simulink model "aaaqi"  (R2016b)
settings: Solver=ode4  StartTime=0.0  StopTime=inf  FixedStep=0.002  RelTol=1e-3  EnableMultiTasking=on
undefined symbols (not defined in the file or in its folder): bit, mdaadlink6208, sigbuilder_block, Standard
libraries: slrtlib x20, slrtsoftinglib x11, simulink x10
(part 1 of 4)
settings Model: xpc_rtwmakecfg_data=_xpccanac2pci_  SimulationMode=external  Creator=Administrator  LastModifiedBy=Administrator
settings SolverCC: EnableConcurrentExecution=on
settings DataIOCC: SaveFormat=StructureWithTime
settings OptimizationCC: BlockReduction=off  OptimizeBlockIOStorage=off  BufferReuse=off  GlobalBufferReuse=off  ExpressionFolding=off  LocalBlockOutputs=off
settings HardwareCC: ProdBitPerPointer=32  ProdBitPerSizeT=32  ProdBitPerPtrDiffT=32  ProdLargestAtomicFloat=None  ProdWordSize=32  ProdLongLongMode=on  ProdHWDeviceType=Generic->32-bit x86 compatible
settings RTWCC: SystemTargetFile=slrt.tlc  TemplateMakefile=slrt_default_tmf  Description=Simulink Real-Time  RTWCompilerOptimization=on

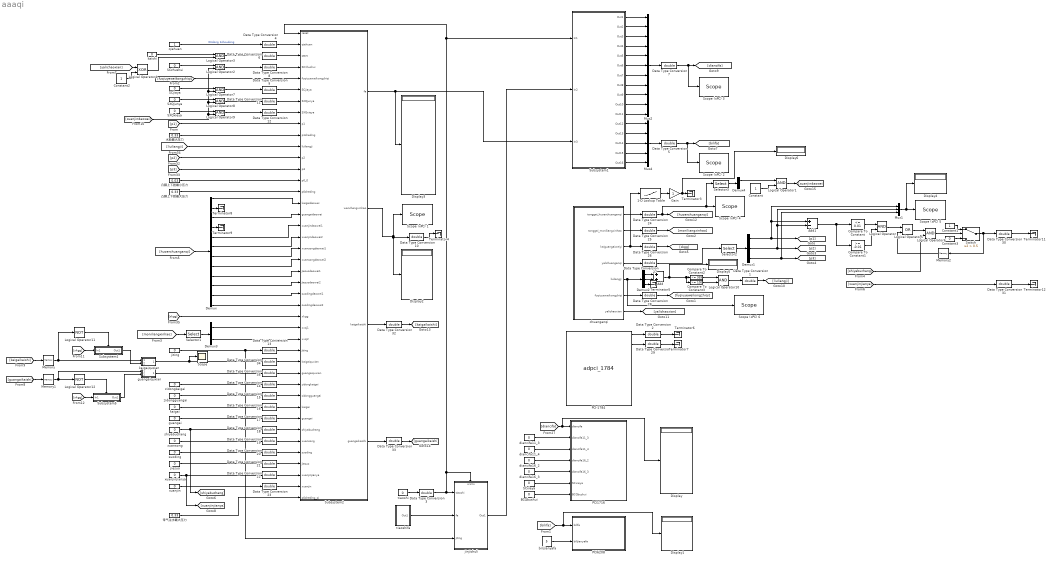
== system aaaqi ==
  1-D Lookup Table : Lookup_n-D  NumberOfTableDimensions=1  BreakpointsForDimension1=[0 600]  Table=[0 115]  InternalRulePriority=Speed  RndMeth=Simplest  InputSameDT=on
  Add : Sum
  Add1 : Sum  Inputs=+-
  BCQbushui : Constant  Value=0
      settings: OpenFcn=|
      | if get_param(gcb,'value')=='1',
      | set_param(gcb,'value','0');
      | else
      | set_param(gcb,'value','1');end
  Compare To Constant : simulink/Logic and Bit Operations/Compare To Constant  relop=<=  const=0.01  OutDataTypeStr=boolean
  Compare To Constant1 : simulink/Logic and Bit Operations/Compare To Constant  relop=>=  const=-0.01  OutDataTypeStr=boolean
  Compare To Constant2 : simulink/Logic and Bit Operations/Compare To Constant  relop=<=  const=999  OutDataTypeStr=boolean
  Compare To Constant3 : simulink/Logic and Bit Operations/Compare To Constant  relop=>=  const=100  OutDataTypeStr=boolean
  Constant : Constant
  Constant1 : Constant
  Constant2 : Constant
  Constant3 : Constant  Value=0
  Data Type Conversion{1..35} (35 alike) : DataTypeConversion  OutDataTypeStr=double
  Demux : Demux  Outputs=12
  Demux1 : Demux  Outputs=3
  Demux2 : Demux  Outputs=3
  Demux3 : Demux  Outputs=2
  Demux4 : Demux  Outputs=2
  Display{,1..6} (7 alike) : Display
  Gain : Gain
  Logical Operator{,1..3,6..10} (9 alike) : Logic  AllPortsSameDT=off  OutDataTypeStr=boolean
  Logical Operator11 : Logic  Operator=NOT  AllPortsSameDT=off  OutDataTypeStr=boolean
  Logical Operator12 : Logic  Operator=NOT  AllPortsSameDT=off  OutDataTypeStr=boolean
  Logical Operator4 : Logic  Operator=XOR  AllPortsSameDT=off  OutDataTypeStr=boolean
  Logical Operator5 : Logic  Operator=OR  AllPortsSameDT=off  OutDataTypeStr=boolean
  Memory : Memory
  Memory1 : Memory
  Memory2 : Memory
  Mux1 : Mux  Inputs=3
  Mux2 : Mux  Inputs=11
  Mux4 : Mux  Inputs=5
  PCI-1784 : S-Function  FunctionName=adpci_1784  Parameters=channel, sampletime, slot  SFunctionDeploymentMode=off  EnableBusSupport=off  mask(PCI-1784){channel=[1 2 3 4 5 6 7 8], sampletime=-1, slot=-1}
      mask prompts: channel "Channel vector:"; sampletime "Sample time:"; slot "PCI slot:"
      mask help:
      | YANHUA
      | PCI-1784
      | Motor Counter
      | UESTC
      mask init:
      | [maskdisplay] = mCntPCI_1784(channel, slot);
      | set_param( gcb, 'MaskDisplay', maskdisplay );
      settings: CopyFcn=|
      | if ~strcmp(get_param(gcb,'Linkstatus'),'none') && ...
      | ~strcmp(get_param(gcb,'Linkstatus'),'implicit')
      |   set_param(gcb,'LinkStatus','none');
      | end
      mask Display: disp('PCI-1784\nUESTC\nMotor Counter');port_label('output',1,'Cnt1');port_label('output',2,'Cnt2');port_label('output',3,'Cnt3');port_label('output',4,'Cnt4');port_label('output',5,'Index1');port_label('output',6,'Index2');port_label('output',7,'Index3');port_label('output',8,'Index4');
  PCI1716 : Subsystem
  PCI6208 : Subsystem
  SCjiaya : Constant  Value=0
      settings: OpenFcn=|
      | if get_param(gcb,'value')=='1',
      | set_param(gcb,'value','0');
      | else
      | set_param(gcb,'value','1');end
  SCxieya : Constant  Value=0
      settings: OpenFcn=|
      | if get_param(gcb,'value')=='1',
      | set_param(gcb,'value','0');
      | else
      | set_param(gcb,'value','1');end
  SCzhushui : Constant  Value=0
      settings: OpenFcn=|
      | if get_param(gcb,'value')=='1',
      | set_param(gcb,'value','0');
      | else
      | set_param(gcb,'value','1');end
  SXQjunya : Constant  Value=0
      settings: OpenFcn=|
      | if get_param(gcb,'value')=='1',
      | set_param(gcb,'value','0');
      | else
      | set_param(gcb,'value','1');end
  SXQxieya : Constant  Value=0
      settings: OpenFcn=|
      | if get_param(gcb,'value')=='1',
      | set_param(gcb,'value','0');
      | else
      | set_param(gcb,'value','1');end
  Scope : Scope
  Scope (xPC) 1 : slrtlib/Displays and Logging/Scope   scopeno=3  scopetype=Target  autostart=on  viewmode=Numerical  formatstr='%15.6f'  grid=on  ylimits=[0,0]  nosamples=250  noprepostsamples=0  interleave=1  triggermode=FreeRun  triggersignal=1  trigsignalfromport=off  triggerlevel=0.0  triggerslope=Either  triggerscope=1  triggersample=0  filename=data.dat  mode=Lazy  writesize=512  autorestart=off  dynamicfilemode=off  maxwritefilesize=512*1024^2
  Scope (xPC) 2 : slrtlib/Displays and Logging/Scope   scopeno=1  scopetype=Target  autostart=on  viewmode=Numerical  formatstr='%15.6f'  grid=on  ylimits=[0,0]  nosamples=250  noprepostsamples=0  interleave=1  triggermode=FreeRun  triggersignal=1  trigsignalfromport=off  triggerlevel=0.0  triggerslope=Either  triggerscope=1  triggersample=0  filename=data.dat  mode=Lazy  writesize=512  autorestart=off  dynamicfilemode=off  maxwritefilesize=512*1024^2
  Scope (xPC) 3 : slrtlib/Displays and Logging/Scope   scopeno=2  scopetype=Target  autostart=on  viewmode=Numerical  formatstr='%15.6f'  grid=on  ylimits=[0,0]  nosamples=250  noprepostsamples=0  interleave=1  triggermode=FreeRun  triggersignal=1  trigsignalfromport=off  triggerlevel=0.0  triggerslope=Either  triggerscope=1  triggersample=0  filename=data.dat  mode=Lazy  writesize=512  autorestart=off  dynamicfilemode=off  maxwritefilesize=512*1024^2
  Scope (xPC) 4 : slrtlib/Displays and Logging/Scope   scopeno=4  scopetype=Target  autostart=on  viewmode=Numerical  formatstr='%15.6f'  grid=on  ylimits=[0,0]  nosamples=250  noprepostsamples=0  interleave=1  triggermode=FreeRun  triggersignal=1  trigsignalfromport=off  triggerlevel=0.0  triggerslope=Either  triggerscope=1  triggersample=0  filename=data.dat  mode=Lazy  writesize=512  autorestart=off  dynamicfilemode=off  maxwritefilesize=512*1024^2
  Scope (xPC) 5 : slrtlib/Displays and Logging/Scope   scopeno=6  scopetype=Target  autostart=on  viewmode=Numerical  formatstr='%15.6f'  grid=on  ylimits=[0,0]  nosamples=250  noprepostsamples=0  interleave=1  triggermode=FreeRun  triggersignal=1  trigsignalfromport=off  triggerlevel=0.0  triggerslope=Either  triggerscope=1  triggersample=0  filename=data.dat  mode=Lazy  writesize=512  autorestart=off  dynamicfilemode=off  maxwritefilesize=512*1024^2
  Scope (xPC) 6 : slrtlib/Displays and Logging/Scope   scopeno=7  scopetype=Target  autostart=on  viewmode=Numerical  formatstr='%15.6f'  grid=on  ylimits=[0,0]  nosamples=250  noprepostsamples=0  interleave=1  triggermode=FreeRun  triggersignal=1  trigsignalfromport=off  triggerlevel=0.0  triggerslope=Either  triggerscope=1  triggersample=0  filename=data.dat  mode=Lazy  writesize=512  autorestart=off  dynamicfilemode=off  maxwritefilesize=512*1024^2
  Selector1 : Selector  IndexOptions=Index vector (dialog)  Indices=[3:4]  OutputSizes=[(-2)]
  Selector2 : Selector  IndexOptions=Index vector (dialog)  Indices=[1 3 5]  OutputSizes=[(-2)]
  Selector3 : Selector  IndexOptions=Index vector (dialog)  Indices=[5 6]  OutputSizes=[(-2)]
  Subsystem1 : Subsystem
  Subsystem2 : Subsystem
  Subsystem4 : Subsystem
  Subsystem5 : Subsystem
  Switch : Switch  Criteria=u2 > Threshold  Threshold=0.5
  Terminator{3..9,11..12} (9 alike) : Terminator
  bilijianyafa : Constant  Value=5
  chuanganqi : Subsystem
  diancifa11_3 : Constant  Value=0
      settings: OpenFcn=|
      | if get_param(gcb,'value')=='1',
      | set_param(gcb,'value','0');
      | else
      | set_param(gcb,'value','1');end
  diancifa11_4 : Constant  Value=0
      settings: OpenFcn=|
      | if get_param(gcb,'value')=='1',
      | set_param(gcb,'value','0');
      | else
      | set_param(gcb,'value','1');end
  diancifa16_2 : Constant  Value=0
      settings: OpenFcn=|
      | if get_param(gcb,'value')=='1',
      | set_param(gcb,'value','0');
      | else
      | set_param(gcb,'value','1');end
  diancifa16_3 : Constant  Value=0
      settings: OpenFcn=|
      | if get_param(gcb,'value')=='1',
      | set_param(gcb,'value','0');
      | else
      | set_param(gcb,'value','1');end
  guangai : Constant  Value=0
      settings: OpenFcn=|
      | if get_param(gcb,'value')=='1',
      | set_param(gcb,'value','0');
      | else
      | set_param(gcb,'value','1');end
  guangaiquxian : Subsystem
  jiesuo : Constant  Value=0
      settings: OpenFcn=|
      | if get_param(gcb,'value')=='1',
      | set_param(gcb,'value','0');
      | else
      | set_param(gcb,'value','1');end
  jinjichuli : Subsystem
  jiting : Constant  Value=0
      settings: OpenFcn=|
      | if get_param(gcb,'value')=='1',
      | set_param(gcb,'value','0');
      | else
      | set_param(gcb,'value','1');end
  kaigai : Constant  Value=0
      settings: OpenFcn=|
      | if get_param(gcb,'value')=='1',
      | set_param(gcb,'value','0');
      | else
      | set_param(gcb,'value','1');end
  kaigaiquxian : Subsystem
  kaishi : Constant  Value=0
      settings: OpenFcn=|
      | if get_param(gcb,'value')=='1',
      | set_param(gcb,'value','0');
      | else
      | set_param(gcb,'value','1');end
  qiehuan : Constant
      settings: OpenFcn=|
      | if get_param(gcb,'value')=='1',
      | set_param(gcb,'value','0');
      | else
      | set_param(gcb,'value','1');end
  shiyabuchang : Constant  Value=0
      settings: OpenFcn=|
      | if get_param(gcb,'value')=='1',
      | set_param(gcb,'value','0');
      | else
      | set_param(gcb,'value','1');end
  suoding : Constant  Value=0
      settings: OpenFcn=|
      | if get_param(gcb,'value')=='1',
      | set_param(gcb,'value','0');
      | else
      | set_param(gcb,'value','1');end
  tiaoshi : Constant  Value=0
      settings: OpenFcn=|
      | if get_param(gcb,'value')=='1',
      | set_param(gcb,'value','0');
      | else
      | set_param(gcb,'value','1');end
  tiaoshifa : Subsystem
  xuanjin : Constant  Value=0
      settings: OpenFcn=|
      | if get_param(gcb,'value')=='1',
      | set_param(gcb,'value','0');
      | else
      | set_param(gcb,'value','1');end
  xuanjinjianya : Constant  Value=0
      settings: OpenFcn=|
      | if get_param(gcb,'value')=='1',
      | set_param(gcb,'value','0');
      | else
      | set_param(gcb,'value','1');end
  xuansong : Constant  Value=0
      settings: OpenFcn=|
      | if get_param(gcb,'value')=='1',
      | set_param(gcb,'value','0');
      | else
      | set_param(gcb,'value','1');end
  zidongguangai : Constant  Value=0
      settings: OpenFcn=|
      | if get_param(gcb,'value')=='1',
      | set_param(gcb,'value','0');
      | else
      | set_param(gcb,'value','1');end
  zidongkaigai : Constant  Value=0
      settings: OpenFcn=|
      | if get_param(gcb,'value')=='1',
      | set_param(gcb,'value','0');
      | else
      | set_param(gcb,'value','1');end
  凸膜上下腔最大压力 : Constant  Value=0.33
  凸膜上下腔最小压力 : Constant  Value=0.03
  带气注水最大压力 : Constant  Value=0.33
  水舱最大压力 : Constant  Value=0.33
  wires:
  jinjichuli/1(Out1) -> Subsystem1/2(In2)
  Mux4/1 -> Data Type Conversion5/1
  qiehuan/1 -> Data Type Conversion4/1  "0zidong 1shoudong"
  SCjiaya/1 -> Logical Operator7/1
  SXQjunya/1 -> Logical Operator8/1
  SXQxieya/1 -> Logical Operator9/1
  水舱最大压力/1 -> Subsystem2/10(p1sheding)
  凸膜上下腔最小压力/1 -> Subsystem2/14(p0_0)
  凸膜上下腔最大压力/1 -> Subsystem2/15(p0sheding)
  zidongkaigai/1 -> Data Type Conversion14/1
  zidongguangai/1 -> Data Type Conversion15/1
  Mux2/1 -> Data Type Conversion7/1
  [diancifa] -> PCI1716/1(diancifa), Display/1
  [p1] -> Subsystem2/9(p1)
  [p2] -> Subsystem2/12(p2)
  [p3] -> Subsystem2/13(p3)
  [huoerchuanganqi] -> Demux/1
  Subsystem2/1(fa) -> Subsystem1/3(In3), Display3/1
  jiting/1 -> jinjichuli/3(jiting), Data Type Conversion13/1
  Subsystem2/2(wanchengxinhao) -> Data Type Conversion10/1, Display2/1, Scope (xPC) 1/1
  Subsystem1/1(Out1) -> Mux2/1
  Subsystem1/2(Out2) -> Mux2/2
  Subsystem1/3(Out3) -> Mux2/3
  Subsystem1/4(Out4) -> Mux2/4
  Subsystem1/5(Out5) -> Mux2/5
  Subsystem1/6(Out6) -> Mux2/6
  Subsystem1/7(Out7) -> Mux2/7
  Subsystem1/8(Out8) -> Mux2/8
  Subsystem1/9(Out9) -> Mux2/9
  tiaoshi/1 -> Data Type Conversion3/1
  [bilifa] -> Display1/1, PCI6208/1(bilifa)
  chuanganqi/4(yalichuanganqi) -> Data Type Conversion27/1
  chuanganqi/1(tonggai_huoerchuanganqi) -> Data Type Conversion24/1
  chuanganqi/6(fuqiuyeweikongzhiqi) -> Data Type Conversion28/1
  SCzhushui/1 -> Logical Operator2/1
  Compare To Constant2/1 -> Logical Operator10/1
  chuanganqi/5(liuliangji) -> Scope (xPC) 6/1, Demux2/1
  Demux2/3 -> Terminator5/1
  Data Type Conversion1/1 -> [liuliangji]
  chuanganqi/3(kaiguangaiweiyi) -> 1-D Lookup Table/1, Data Type Conversion26/1
  PCI-1784/1 -> Data Type Conversion2/1
  Data Type Conversion2/1 -> Terminator6/1
  shiyabuchang/1 -> [shiyabuchang], Data Type Conversion18/1
  suoding/1 -> Data Type Conversion20/1
  jiesuo/1 -> Data Type Conversion21/1
  xuanjinjianya/1 -> [xuanjinjianya], Data Type Conversion22/1
  tiaoshifa/1(Out1) -> jinjichuli/2(fa)
  Data Type Conversion3/1 -> jinjichuli/1(tiaoshi), jinjichuli/Enable, Subsystem2/1(reset), Subsystem1/1(In1)
  Data Type Conversion4/1 -> Subsystem2/2(qiehuan)
  Data Type Conversion6/1 -> Subsystem2/3(start)
  Data Type Conversion8/1 -> Subsystem2/4(SCzhushui)
  Data Type Conversion9/1 -> Subsystem2/6(SCjiaya)
  Data Type Conversion11/1 -> Subsystem2/7(SXQjunya)
  Data Type Conversion12/1 -> Subsystem2/8(SXQxieya)
  Data Type Conversion13/1 -> Subsystem2/29(jiting)
  Data Type Conversion14/1 -> Subsystem2/32(zidongkaigai)
  Data Type Conversion15/1 -> Subsystem2/33(zidongguangai)
  Data Type Conversion18/1 -> Subsystem2/36(shiyabuchang)
  Data Type Conversion22/1 -> Subsystem2/40(xuanjinjianya)
  Data Type Conversion7/1 -> Scope (xPC) 3/1, [diancifa]
  Data Type Conversion5/1 -> [bilifa], Scope (xPC) 2/1
  chuanganqi/2(tonggai_moniliangxinhao) -> Data Type Conversion25/1
  Data Type Conversion26/1 -> [xkgg]
  Data Type Conversion27/1 -> Selector2/1
  Data Type Conversion28/1 -> [fuqiuyeweikongzhiqi]
  Data Type Conversion25/1 -> [moniliangxinhao]
  Data Type Conversion29/1 -> Terminator7/1
  PCI-1784/2 -> Data Type Conversion29/1
  [moniliangxinhao] -> Selector1/1
  Selector1/1 -> Demux3/1
  Demux3/1 -> Subsystem2/27(xxsj1)
  Demux3/2 -> Subsystem2/28(xxsj2)
  Subsystem1/11(Out11) -> Mux2/11
  Subsystem1/10(Out10) -> Mux2/10
  Subsystem1/12(Out12) -> Mux4/1
  Subsystem1/13(Out13) -> Mux4/2
  Subsystem1/14(Out14) -> Mux4/3
  Subsystem1/15(Out15) -> Mux4/4
  Subsystem1/16(Out16) -> Mux4/5
  Demux/2 -> Terminator8/1
  Demux/4 -> Terminator9/1
  Demux/12 -> Subsystem2/25(suodingdaowei2)
  Demux/11 -> Subsystem2/24(suodingdaowei1)
  Demux/10 -> Subsystem2/23(jiesuodaowei2)
  Demux/3 -> Subsystem2/17(guangaidaowei)
  Demux/9 -> Subsystem2/22(jiesuodaowei1)
  Demux/1 -> Subsystem2/16(kaigaidaowei)
  Demux/8 -> Subsystem2/21(xuansongdaowei2)
  Demux/7 -> Subsystem2/20(xuansongdaowei1)
  Demux/6 -> Subsystem2/19(xuanjindaowei2)
  Demux/5 -> Subsystem2/18(xuanjindaowei1)
  Demux2/1 -> Add/1
  Demux2/2 -> Add/2
  Add/1 -> Display5/1, Compare To Constant3/1, Compare To Constant2/1
  [fuqiuyeweikongzhiqi] -> Subsystem2/5(fuqiuyeweikongzhiqi)
  [liuliangji] -> Subsystem2/11(liuliangji)
  diancifa11_4/1 -> PCI1716/3(diancifa11_4)
  diancifa16_2/1 -> PCI1716/4(diancifa16_2)
  diancifa16_3/1 -> PCI1716/5(diancifa16_3)
  Demux1/2 -> Add1/2, Mux1/2, [p2]
  Demux1/1 -> Mux1/1, Add1/1, [p1]
  Demux1/3 -> Mux1/3, [p3]
  Data Type Conversion10/1 -> Terminator4/1
  Mux1/1 -> Display4/1, Scope (xPC) 5/1
  Add1/1 -> Compare To Constant/1, Compare To Constant1/1
  Compare To Constant/1 -> Logical Operator/1
  Compare To Constant1/1 -> Logical Operator/2
  Data Type Conversion30/1 -> Terminator11/1
  Logical Operator/1 -> Logical Operator5/1
  [shiyabuchang] -> Logical Operator6/2
  Data Type Conversion31/1 -> Terminator12/1
  [xuanjinjianya] -> Data Type Conversion31/1
  diancifa11_3/1 -> PCI1716/2(diancifa11_3)
  bilijianyafa/1 -> PCI6208/2(bilijianyafa)
  chuanganqi/7(yalichaoxian) -> [yalichaoxian]
  Logical Operator3/1 -> Data Type Conversion6/1
  kaishi/1 -> Logical Operator3/1
  Constant2/1 -> Logical Operator4/2
  [yalichaoxian] -> Logical Operator4/1
  Logical Operator4/1 -> Logical Operator3/2
  SCxieya/1 -> PCI1716/6(SCxieya)
  BCQbushui/1 -> PCI1716/7(BCQbushui)
  Data Type Conversion32/1 -> [kaigaikaishi]
  Subsystem2/3(kaigaikaishi) -> Data Type Conversion32/1
  Data Type Conversion33/1 -> [guangaikaishi]
  Subsystem2/4(guangaikaishi) -> Data Type Conversion33/1
  kaigaiquxian/1(Out1) -> Scope/1, Data Type Conversion34/1
  guangaiquxian/1(Out1) -> Data Type Conversion35/1
  [guangaikaishi] -> Memory1/1
  Data Type Conversion34/1 -> Subsystem2/30(kaigaiquxian)
  Data Type Conversion35/1 -> Subsystem2/31(guangaiquxian)
  Memory/1 -> Logical Operator11/1, kaigaiquxian/1(In1)
  Logical Operator5/1 -> Logical Operator6/1
  Logical Operator6/1 -> Switch/2
  Constant1/1 -> Switch/1
  Constant3/1 -> Switch/3
  Switch/1 -> Memory2/1, Data Type Conversion30/1
  Memory2/1 -> Logical Operator5/2
  Data Type Conversion17/1 -> Subsystem2/35(guangai)
  Data Type Conversion16/1 -> Subsystem2/34(kaigai)
  Data Type Conversion21/1 -> Subsystem2/39(jiesuo)
  Data Type Conversion20/1 -> Subsystem2/38(suoding)
  Data Type Conversion19/1 -> Subsystem2/37(xuansong)
  Data Type Conversion23/1 -> Subsystem2/41(xuanjin)
  1-D Lookup Table/1 -> Gain/1
  Gain/1 -> Display6/1, Terminator3/1
  Data Type Conversion24/1 -> Selector3/1, Scope (xPC) 4/1, [huoerchuanganqi]
  Selector3/1 -> Demux4/1
  Demux4/1 -> Logical Operator1/1
  Logical Operator1/1 -> [xuanjindaowei]
  Logical Operator2/1 -> Data Type Conversion8/1
  Logical Operator7/1 -> Data Type Conversion9/1
  Logical Operator8/1 -> Data Type Conversion11/1
  Logical Operator9/1 -> Data Type Conversion12/1
  [xuanjindaowei] -> Logical Operator2/2, Logical Operator7/2, Logical Operator8/2, Logical Operator9/2
  Selector2/1 -> Demux1/1
  Compare To Constant3/1 -> Logical Operator10/2
  Logical Operator10/1 -> Data Type Conversion1/1
  [xkgg] -> Subsystem4/1(In1)
  Logical Operator11/1 -> Subsystem4/Enable
  Subsystem4/1(Out1) -> kaigaiquxian/2(In2)
  Memory1/1 -> guangaiquxian/1(In1), Logical Operator12/1
  [xkgg] -> Subsystem5/1(In1)
  Logical Operator12/1 -> Subsystem5/Enable
  Subsystem5/1(Out1) -> guangaiquxian/2(In2)
  [kaigaikaishi] -> Memory/1
  xuanjin/1 -> Data Type Conversion23/1
  xuansong/1 -> Data Type Conversion19/1
  kaigai/1 -> Data Type Conversion16/1
  guangai/1 -> Data Type Conversion17/1
  [xkgg] -> Subsystem2/26(xkgg)
  带气注水最大压力/1 -> Subsystem2/42(p0sheding_qi)
  Constant/1 -> Logical Operator1/2

== system aaaqi/PCI1716 ==
  diancifa : Inport
  diancifa11_3 : Inport  Port=2
  diancifa11_4 : Inport  Port=3
  diancifa16_2 : Inport  Port=4
  diancifa16_3 : Inport  Port=5
  SCxieya : Inport  Port=6
  BCQbushui : Inport  Port=7
  Data Type Conversion : DataTypeConversion  OutDataTypeStr=double
  Data Type Conversion1 : DataTypeConversion  OutDataTypeStr=double
  Data Type Conversion2 : DataTypeConversion  OutDataTypeStr=double
  Demux : Demux  Outputs=11
  Logical Operator : Logic  Operator=OR  AllPortsSameDT=off  OutDataTypeStr=boolean
  Logical Operator1 : Logic  Operator=OR  AllPortsSameDT=off  OutDataTypeStr=boolean
  Mux : Mux  Inputs=15
  PCI1716DIO1 : S-Function  FunctionName=pci1716DIO  Parameters=[SampleTime SampleOffset], SLOT  SFunctionDeploymentMode=off  EnableBusSupport=off  mask{Sample=-1, SLOT=-1}
      mask prompts: Sample "Sample Time:"
      mask help:
      | PCI1716DIO
      | A/D Card
      | Harbin
      | 2014.06.06
      mask init:
      | SampleTime = -1; SampleOffset=0;
      mask Display:
      | disp('PCI1716   A/D&D/A&DIO  ');
      | port_label('input',1 , 'IN1');
      | port_label('input',2 , 'IN2');
      | port_label('input',3 , 'D1');
      | port_label('input',4 , 'D2');
      | port_label('input',5 , 'D3');
      | port_label('input',6 , 'D4');
      | port_label('input',7 , 'D5');
      | port_label('input',8 , 'D6');
      | port_label('input',9 , 'D7');
      | port_label('input',10 , 'D8');
      | port_label('input',11 , 'D9');
      | port_label('input',12 , 'D10');
      | port_label('input',13 , 'D11');
      | port_label('input',14 , 'D12');
      | port_label('input',15 , 'D13');
      | port_label('input',16 , 'D14');
      | port_label('input',17 , 'D15');
      | port_label('input',18, 'D16');
      | port_label('output',1 , 'AD(16)');
      | port_label('output',2 , 'D_OUT(16)');
  Terminator : Terminator
  constant : Constant  Value=0
      settings: OpenFcn=|
      | if get_param(gcb,'value')=='1',
      | set_param(gcb,'value','0');
      | else
      | set_param(gcb,'value','1');end
  wires:
  diancifa/1 -> Demux/1
  Demux/2 -> PCI1716DIO1/4, Mux/2  "diancifa11_2"
  Demux/10 -> Mux/14, PCI1716DIO1/17  "xuansong"
  Demux/3 -> PCI1716DIO1/7, Mux/5  "diancifa11_5"
  Demux/4 -> PCI1716DIO1/12, Mux/9  "diancifa20"
  Demux/6 -> PCI1716DIO1/11, Mux/11  "diancifa3"
  Demux/7 -> Logical Operator1/1  "diancifa21"
  Demux/8 -> PCI1716DIO1/15, Mux/12  "suoding"
  Demux/9 -> PCI1716DIO1/16, Mux/13  "jiesuo"
  diancifa11_4/1 -> Mux/4, PCI1716DIO1/6
  diancifa16_2/1 -> Mux/7, PCI1716DIO1/9
  diancifa16_3/1 -> Mux/8, PCI1716DIO1/10
  Demux/1 -> PCI1716DIO1/3, Mux/1  "diancifa11_1"
  constant/1 -> PCI1716DIO1/14
  Demux/11 -> PCI1716DIO1/18, Mux/15  "xuanjin"
  diancifa11_3/1 -> Mux/3, PCI1716DIO1/5
  SCxieya/1 -> Logical Operator/2
  Demux/5 -> Logical Operator/1  "diancifa16_1"
  Logical Operator/1 -> Data Type Conversion1/1
  Data Type Conversion1/1 -> Mux/6, PCI1716DIO1/8
  Mux/1 -> Data Type Conversion/1
  Data Type Conversion/1 -> Terminator/1
  Logical Operator1/1 -> Data Type Conversion2/1
  BCQbushui/1 -> Logical Operator1/2
  Data Type Conversion2/1 -> Mux/10, PCI1716DIO1/13

== system aaaqi/PCI6208 ==
  bilifa : Inport
  bilijianyafa : Inport  Port=2
  Constant : Constant  Value=0
  Constant1 : Constant  Value=0
  Data Type Conversion : DataTypeConversion  OutDataTypeStr=double
  Demux : Demux  Outputs=5
  "PCI-6208A DA " : S-Function  InitFcn=mdaadlink6208( 1 );  FunctionName=da6208  Parameters=channel, range, sampletime, pcislot, reset, initval  SFunctionDeploymentMode=off  EnableBusSupport=off  mask(da6208){channel=[1:8], range=4 to 20 ma, reset=[0], initval=[0], sampletime=-1, pcislot=-1}
      mask prompts: channel "Channel vector:"; reset "Reset vector:"; initval "Initial value vector:"; sampletime "Sample time:"; pcislot "PCI slot (-1: autosearch):"
      mask help:
      | PCI-6208A
      | Adlink
      | Analog Output
      mask init:
      | [maskdisplay, reset, initval]= mdaadlink6208(2, channel, reset, initval, pcislot);
      | set_param(gcb,'MaskDisplay',maskdisplay);
      mask Help: helpview(fullfile(docroot, 'mapfiles', 'xpc.map'), 'Adlink_6208A_DA')
      mask TypeOptions range: 0 to 20 ma | 5 to 25 ma | 4 to 20 ma
      mask Display: disp('PCI-6208A\nAdlink\nAnalog Output');port_label('input',1,'1');port_label('input',2,'2');port_label('input',3,'3');port_label('input',4,'4');port_label('input',5,'5');port_label('input',6,'6');port_label('input',7,'7');port_label('input',8,'8');
  Saturation{,1..3,7} (5 alike) : Saturate  UpperLimit=10  LowerLimit=0
  Saturation4 : Saturate  UpperLimit=10  LowerLimit=-10
  Saturation5 : Saturate  UpperLimit=10  LowerLimit=-10
  Saturation6 : Saturate  UpperLimit=10  LowerLimit=-10
  wires:
  bilifa/1 -> Data Type Conversion/1
  Demux/1 -> Saturation/1  "18.1"
  Demux/2 -> Saturation1/1  "18.2"
  Demux/3 -> Saturation2/1  "18.3"
  Demux/4 -> Saturation3/1  "18.4"
  Demux/5 -> Saturation4/1  "kaiguangaibilihuanxiangfa"
  Constant/1 -> Saturation5/1
  bilijianyafa/1 -> Saturation7/1
  Constant1/1 -> Saturation6/1
  Saturation/1 -> "PCI-6208A DA "/1
  Saturation1/1 -> "PCI-6208A DA "/2
  Saturation2/1 -> "PCI-6208A DA "/3
  Saturation3/1 -> "PCI-6208A DA "/4
  Saturation4/1 -> "PCI-6208A DA "/5
  Saturation5/1 -> "PCI-6208A DA "/6
  Saturation6/1 -> "PCI-6208A DA "/7
  Saturation7/1 -> "PCI-6208A DA "/8
  Data Type Conversion/1 -> Demux/1

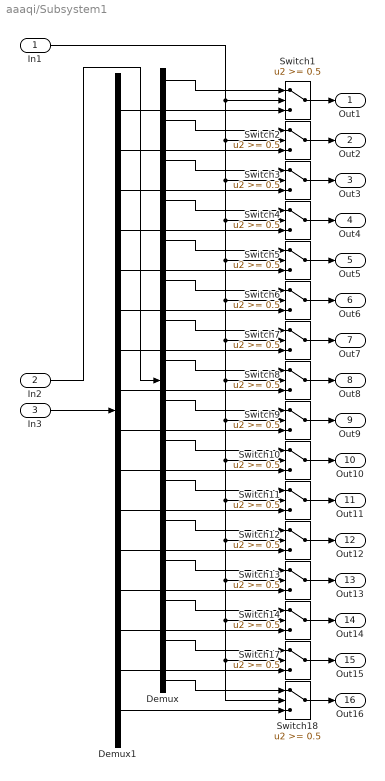
== system aaaqi/Subsystem1 ==
  In1 : Inport
  In2 : Inport  Port=2
  In3 : Inport  Port=3
  Demux : Demux  Outputs=16
  Demux1 : Demux  Outputs=16
  Switch{1..14,17..18} (16 alike) : Switch  Threshold=0.5  SaturateOnIntegerOverflow=on
  Out1 : Outport
  Out2 : Outport  Port=2
  Out3 : Outport  Port=3
  Out4 : Outport  Port=4
  Out5 : Outport  Port=5
  Out6 : Outport  Port=6
  Out7 : Outport  Port=7
  Out8 : Outport  Port=8
  Out9 : Outport  Port=9
  Out10 : Outport  Port=10
  Out11 : Outport  Port=11
  Out12 : Outport  Port=12
  Out13 : Outport  Port=13
  Out14 : Outport  Port=14
  Out15 : Outport  Port=15
  Out16 : Outport  Port=16
  wires:
  Switch1/1 -> Out1/1
  Switch2/1 -> Out2/1
  Switch3/1 -> Out3/1
  Switch4/1 -> Out4/1
  Switch5/1 -> Out5/1
  Switch6/1 -> Out6/1
  Switch7/1 -> Out7/1
  Switch8/1 -> Out8/1
  Switch9/1 -> Out9/1
  Switch10/1 -> Out10/1
  Switch11/1 -> Out11/1
  Switch12/1 -> Out12/1
  Switch13/1 -> Out13/1
  Switch14/1 -> Out14/1
  Switch17/1 -> Out15/1
  Switch18/1 -> Out16/1
  Demux/1 -> Switch1/1
  Demux/2 -> Switch2/1
  Demux/3 -> Switch3/1
  Demux/4 -> Switch4/1
  Demux/5 -> Switch5/1
  Demux/6 -> Switch6/1
  Demux/7 -> Switch7/1
  Demux/8 -> Switch8/1
  Demux/9 -> Switch9/1
  Demux/10 -> Switch10/1
  Demux/11 -> Switch11/1
  Demux/12 -> Switch12/1
  Demux/13 -> Switch13/1
  Demux/14 -> Switch14/1
  Demux/15 -> Switch17/1
  Demux/16 -> Switch18/1
  Demux1/1 -> Switch1/3
  Demux1/2 -> Switch2/3
  Demux1/3 -> Switch3/3
  Demux1/4 -> Switch4/3
  Demux1/5 -> Switch5/3
  Demux1/6 -> Switch6/3
  Demux1/7 -> Switch7/3
  Demux1/8 -> Switch8/3
  Demux1/9 -> Switch9/3
  Demux1/10 -> Switch10/3
  Demux1/11 -> Switch11/3
  Demux1/12 -> Switch12/3
  Demux1/13 -> Switch13/3
  Demux1/14 -> Switch14/3
  Demux1/15 -> Switch17/3
  Demux1/16 -> Switch18/3
  In1/1 -> Switch1/2, Switch2/2, Switch3/2, Switch4/2, Switch5/2, Switch6/2, Switch7/2, Switch8/2, Switch9/2, Switch10/2, Switch11/2, Switch12/2, Switch13/2, Switch14/2, Switch17/2, Switch18/2
  In2/1 -> Demux/1
  In3/1 -> Demux1/1

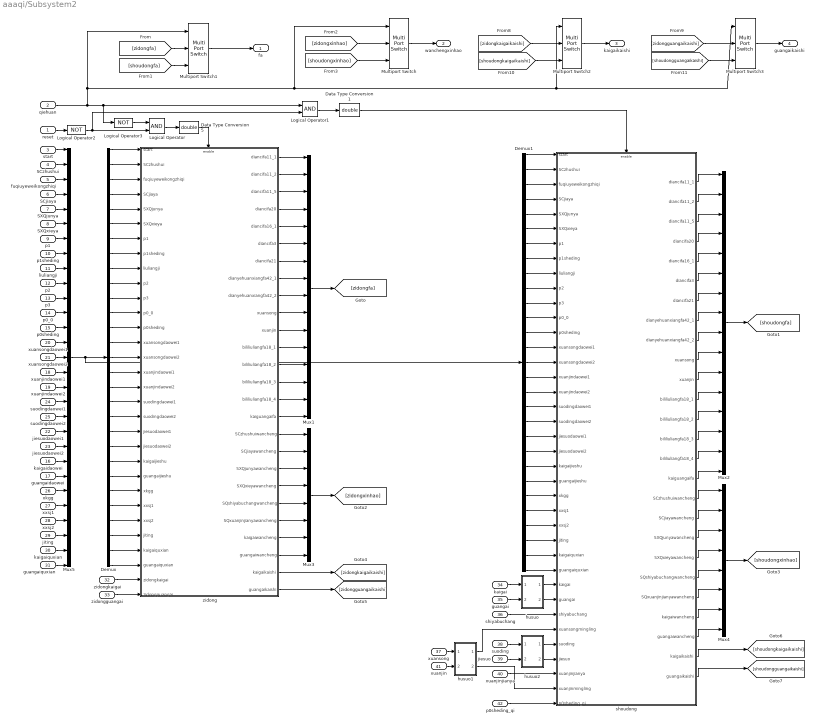
== system aaaqi/Subsystem2 ==
  reset : Inport
  qiehuan : Inport  Port=2
  start : Inport  Port=3
  SCzhushui : Inport  Port=4
  fuqiuyeweikongzhiqi : Inport  Port=5
  SCjiaya : Inport  Port=6
  SXQjunya : Inport  Port=7
  SXQxieya : Inport  Port=8
  p1 : Inport  Port=9
  p1sheding : Inport  Port=10
  liuliangji : Inport  Port=11
  p2 : Inport  Port=12
  p3 : Inport  Port=13
  p0_0 : Inport  Port=14
  p0sheding : Inport  Port=15
  kaigaidaowei : Inport  Port=16
  guangaidaowei : Inport  Port=17
  xuanjindaowei1 : Inport  Port=18
  xuanjindaowei2 : Inport  Port=19
  xuansongdaowei1 : Inport  Port=20
  xuansongdaowei2 : Inport  Port=21
  jiesuodaowei1 : Inport  Port=22
  jiesuodaowei2 : Inport  Port=23
  suodingdaowei1 : Inport  Port=24
  suodingdaowei2 : Inport  Port=25
  xkgg : Inport  Port=26
  xxsj1 : Inport  Port=27
  xxsj2 : Inport  Port=28
  jiting : Inport  Port=29
  kaigaiquxian : Inport  Port=30
  guangaiquxian : Inport  Port=31
  zidongkaigai : Inport  Port=32
  zidongguangai : Inport  Port=33
  kaigai : Inport  Port=34
  guangai : Inport  Port=35
  shiyabuchang : Inport  Port=36
  xuansong : Inport  Port=37
  suoding : Inport  Port=38
  jiesuo : Inport  Port=39
  xuanjinjianya : Inport  Port=40
  xuanjin : Inport  Port=41
  p0sheding_qi : Inport  Port=42
  Data Type Conversion1 : DataTypeConversion  OutDataTypeStr=double
  Data Type Conversion5 : DataTypeConversion  OutDataTypeStr=double
  Demux : Demux  Outputs=29
  Demux1 : Demux  Outputs=29
  Logical Operator : Logic  AllPortsSameDT=off  OutDataTypeStr=boolean
  Logical Operator1 : Logic  AllPortsSameDT=off  OutDataTypeStr=boolean
  Logical Operator2 : Logic  Operator=NOT  AllPortsSameDT=off  OutDataTypeStr=boolean
  Logical Operator3 : Logic  Operator=NOT  AllPortsSameDT=off  OutDataTypeStr=boolean
  Multiport Switch{,1..3} (4 alike) : MultiPortSwitch  DataPortOrder=Zero-based contiguous  Inputs=2  zeroidx=on
  Mux1 : Mux  Inputs=16
  Mux2 : Mux  Inputs=16
  Mux3 : Mux  Inputs=8
  Mux4 : Mux  Inputs=8
  Mux5 : Mux  Inputs=29
  husuo : Subsystem
  husuo1 : Subsystem
  husuo2 : Subsystem
  shoudong : Subsystem
  zidong : Subsystem
  fa : Outport
  wanchengxinhao : Outport  Port=2
  kaigaikaishi : Outport  Port=3
  guangaikaishi : Outport  Port=4
  wires:
  Demux/1 -> zidong/1(start)
  Demux/2 -> zidong/2(SCzhushui)
  Demux/3 -> zidong/3(fuqiuyeweikongzhiqi)
  Demux/4 -> zidong/4(SCjiaya)
  Demux/5 -> zidong/5(SXQjunya)
  Demux/6 -> zidong/6(SXQxieya)
  Demux/7 -> zidong/7(p1)
  Demux/8 -> zidong/8(p1sheding)
  Demux/9 -> zidong/9(liuliangji)
  Demux/10 -> zidong/10(p2)
  Demux/11 -> zidong/11(p3)
  Demux/12 -> zidong/12(p0_0)
  Demux/13 -> zidong/13(p0sheding)
  Mux5/1 -> Demux/1, Demux1/1
  Logical Operator/1 -> Data Type Conversion5/1
  Logical Operator1/1 -> Data Type Conversion1/1
  Data Type Conversion1/1 -> shoudong/Enable
  Logical Operator2/1 -> Logical Operator/2, Logical Operator1/2
  Data Type Conversion5/1 -> zidong/Enable
  reset/1 -> Logical Operator2/1
  zidong/1(diancifa11_1) -> Mux1/1
  zidong/2(diancifa11_2) -> Mux1/2
  zidong/3(diancifa11_5) -> Mux1/3
  zidong/4(diancifa20) -> Mux1/4
  zidong/5(diancifa16_1) -> Mux1/5
  zidong/6(diancifa3) -> Mux1/6
  zidong/7(diancifa21) -> Mux1/7
  start/1 -> Mux5/1
  SCzhushui/1 -> Mux5/2
  fuqiuyeweikongzhiqi/1 -> Mux5/3
  SCjiaya/1 -> Mux5/4
  SXQjunya/1 -> Mux5/5
  SXQxieya/1 -> Mux5/6
  p1sheding/1 -> Mux5/8
  liuliangji/1 -> Mux5/9
  p2/1 -> Mux5/10
  p3/1 -> Mux5/11
  p0_0/1 -> Mux5/12
  p0sheding/1 -> Mux5/13
  Mux1/1 -> [zidongfa]
  p1/1 -> Mux5/7
  zidong/17(SCzhushuiwancheng) -> Mux3/1
  zidong/18(SCjiayawancheng) -> Mux3/2
  zidong/19(SXQjunyawancheng) -> Mux3/3
  zidong/20(SXQxieyawancheng) -> Mux3/4
  zidong/21(SQshiyabuchangwancheng) -> Mux3/5
  zidong/22(SQxuanjinjianyawancheng) -> Mux3/6
  zidong/23(kaigaiwancheng) -> Mux3/7
  zidong/24(guangaiwancheng) -> Mux3/8
  Mux3/1 -> [zidongxinhao]
  [zidongxinhao] -> Multiport Switch/2
  [shoudongxinhao] -> Multiport Switch/3
  Multiport Switch/1 -> wanchengxinhao/1
  zidong/12(bililiuliangfa18_1) -> Mux1/12
  zidong/15(bililiuliangfa18_4) -> Mux1/15
  zidong/16(kaiguangaifa) -> Mux1/16
  Mux2/1 -> [shoudongfa]
  Demux1/1 -> shoudong/1(start)
  Demux1/2 -> shoudong/2(SCzhushui)
  Demux1/3 -> shoudong/3(fuqiuyeweikongzhiqi)
  Demux1/4 -> shoudong/4(SCjiaya)
  Demux1/5 -> shoudong/5(SXQjunya)
  Demux1/6 -> shoudong/6(SXQxieya)
  Demux1/7 -> shoudong/7(p1)
  Demux1/8 -> shoudong/8(p1sheding)
  Demux1/9 -> shoudong/9(liuliangji)
  Demux1/10 -> shoudong/10(p2)
  Demux1/11 -> shoudong/11(p3)
  Demux1/12 -> shoudong/12(p0_0)
  Demux1/13 -> shoudong/13(p0sheding)
  shoudong/1(diancifa11_1) -> Mux2/1
  shoudong/2(diancifa11_2) -> Mux2/2
  shoudong/3(diancifa11_5) -> Mux2/3
  shoudong/4(diancifa20) -> Mux2/4
  shoudong/5(diancifa16_1) -> Mux2/5
  shoudong/6(diancifa3) -> Mux2/6
  shoudong/7(diancifa21) -> Mux2/7
  shoudong/17(SCzhushuiwancheng) -> Mux4/1
  shoudong/18(SCjiayawancheng) -> Mux4/2
  shoudong/19(SXQjunyawancheng) -> Mux4/3
  shoudong/20(SXQxieyawancheng) -> Mux4/4
  shoudong/21(SQshiyabuchangwancheng) -> Mux4/5
  shoudong/22(SQxuanjinjianyawancheng) -> Mux4/6
  shoudong/23(kaigaiwancheng) -> Mux4/7
  shoudong/24(guangaiwancheng) -> Mux4/8
  shoudong/12(bililiuliangfa18_1) -> Mux2/12
  shoudong/15(bililiuliangfa18_4) -> Mux2/15
  shoudong/16(kaiguangaifa) -> Mux2/16
  zidong/13(bililiuliangfa18_2) -> Mux1/13
  zidong/14(bililiuliangfa18_3) -> Mux1/14
  shoudong/13(bililiuliangfa18_2) -> Mux2/13
  shoudong/14(bililiuliangfa18_3) -> Mux2/14
  Demux/14 -> zidong/14(xuansongdaowei1)
  Demux/15 -> zidong/15(xuansongdaowei2)
  Demux/16 -> zidong/16(xuanjindaowei1)
  Demux/17 -> zidong/17(xuanjindaowei2)
  Demux/18 -> zidong/18(suodingdaowei1)
  Demux/19 -> zidong/19(suodingdaowei2)
  Demux/20 -> zidong/20(jiesuodaowei1)
  Demux/21 -> zidong/21(jiesuodaowei2)
  Demux/22 -> zidong/22(kaigaijieshu)
  Demux/23 -> zidong/23(guangaijieshu)
  Demux/24 -> zidong/24(xkgg)
  Demux/27 -> zidong/27(jiting)
  xuansongdaowei1/1 -> Mux5/14
  xuansongdaowei2/1 -> Mux5/15
  xuanjindaowei1/1 -> Mux5/16
  xuanjindaowei2/1 -> Mux5/17
  suodingdaowei1/1 -> Mux5/18
  suodingdaowei2/1 -> Mux5/19
  jiesuodaowei1/1 -> Mux5/20
  jiesuodaowei2/1 -> Mux5/21
  kaigaidaowei/1 -> Mux5/22
  guangaidaowei/1 -> Mux5/23
  xkgg/1 -> Mux5/24
  jiting/1 -> Mux5/27
  zidongkaigai/1 -> zidong/30(zidongkaigai)
  zidongguangai/1 -> zidong/31(zidongguangai)
  Demux1/14 -> shoudong/14(xuansongdaowei1)
  Demux1/15 -> shoudong/15(xuansongdaowei2)
  Demux1/16 -> shoudong/16(xuanjindaowei1)
  Demux1/17 -> shoudong/17(xuanjindaowei2)
  Demux1/18 -> shoudong/18(suodingdaowei1)
  Demux1/19 -> shoudong/19(suodingdaowei2)
  Demux1/20 -> shoudong/20(jiesuodaowei1)
  Demux1/21 -> shoudong/21(jiesuodaowei2)
  Demux1/22 -> shoudong/22(kaigaijieshu)
  Demux1/23 -> shoudong/23(guangaijieshu)
  Demux1/24 -> shoudong/24(xkgg)
  Demux1/27 -> shoudong/27(jiting)
  shiyabuchang/1 -> shoudong/32(shiyabuchang)
  xuanjinjianya/1 -> shoudong/36(xuanjinjianya)
  Demux/25 -> zidong/25(xxsj1)
  Demux/26 -> zidong/26(xxsj2)
  xxsj1/1 -> Mux5/25
  xxsj2/1 -> Mux5/26
  Demux1/25 -> shoudong/25(xxsj1)
  Demux1/26 -> shoudong/26(xxsj2)
  zidong/8(dianyehuanxiangfa42_1) -> Mux1/8
  zidong/10(xuansong) -> Mux1/10
  zidong/11(xuanjin) -> Mux1/11
  shoudong/8(dianyehuanxiangfa42_1) -> Mux2/8
  shoudong/9(dianyehuanxiangfa42_2) -> Mux2/9
  shoudong/10(xuansong) -> Mux2/10
  shoudong/11(xuanjin) -> Mux2/11
  qiehuan/1 -> Logical Operator1/1, Logical Operator3/1, Multiport Switch2/1, Multiport Switch3/1, Multiport Switch/1, Multiport Switch1/1
  Logical Operator3/1 -> Logical Operator/1
  [zidongfa] -> Multiport Switch1/2
  [shoudongfa] -> Multiport Switch1/3
  Mux4/1 -> [shoudongxinhao]
  zidong/9(dianyehuanxiangfa42_2) -> Mux1/9
  Multiport Switch1/1 -> fa/1
  [zidongkaigaikaishi] -> Multiport Switch2/2
  [shoudongkaigaikaishi] -> Multiport Switch2/3
  Multiport Switch2/1 -> kaigaikaishi/1
  [zidongguangaikaishi] -> Multiport Switch3/2
  [shoudongguangaikaishi] -> Multiport Switch3/3
  Multiport Switch3/1 -> guangaikaishi/1
  zidong/25(kaigaikaishi) -> [zidongkaigaikaishi]
  zidong/26(guangaikaishi) -> [zidongguangaikaishi]
  shoudong/25(kaigaikaishi) -> [shoudongkaigaikaishi]
  shoudong/26(guangaikaishi) -> [shoudongguangaikaishi]
  kaigaiquxian/1 -> Mux5/28
  guangaiquxian/1 -> Mux5/29
  Demux/28 -> zidong/28(kaigaiquxian)
  Demux/29 -> zidong/29(guangaiquxian)
  Demux1/28 -> shoudong/28(kaigaiquxian)
  Demux1/29 -> shoudong/29(guangaiquxian)
  husuo/1(Out1) -> shoudong/30(kaigai)
  husuo/2(Out2) -> shoudong/31(guangai)
  kaigai/1 -> husuo/1(In1)
  guangai/1 -> husuo/2(In2)
  xuansong/1 -> husuo1/1(In1)
  xuanjin/1 -> husuo1/2(In2)
  husuo1/1(Out1) -> shoudong/33(xuansongmingling)
  husuo1/2(Out2) -> shoudong/37(xuanjinmingling)
  suoding/1 -> husuo2/1(In1)
  jiesuo/1 -> husuo2/2(In2)
  husuo2/1(Out1) -> shoudong/34(suoding)
  husuo2/2(Out2) -> shoudong/35(jiesuo)
  p0sheding_qi/1 -> shoudong/38(p0sheding_qi)

== system aaaqi/Subsystem4 ==
  In1 : Inport
  Enable : EnablePort
  Add : Sum  Inputs=+-
  Constant : Constant  Value=20
  Out1 : Outport
  wires:
  In1/1 -> Add/1
  Add/1 -> Out1/1
  Constant/1 -> Add/2

== system aaaqi/Subsystem5 ==
  In1 : Inport
  Enable : EnablePort
  Add : Sum  Inputs=+-
  Constant : Constant  Value=600
  Out1 : Outport
  wires:
  Constant/1 -> Add/2
  Add/1 -> Out1/1
  In1/1 -> Add/1
